simulink model "yukti_arduino_comms"  (R2025b)
settings: Solver=ode3  StartTime=0.0  StopTime=10  FixedStep=0.01  RelTol=1e-3  EnableMultiTasking=on
libraries: raspberrypiBasiclib x3, simulink_extras x2, instrumentseriallib x2, slpidlib x1, raspberrypiCommlib x1, raspberrypiNetworklib x1, instrumentlib x1
settings Model: FPTRunName=Active  ExtModeTrigDuration=2  Creator=YuktiVijay  LastModifiedBy=YuktiVijay
settings SolverCC: AlgebraicLoopSolver=TrustRegion  PositivePriorityOrder=on
settings DataIOCC: LimitDataPoints=on  SaveFormat=Array
settings OptimizationCC: ExpressionDepthLimit=2147483647.0  LifeSpan=Inf  MaxStackSize=200000
settings DebuggingCC: UnderspecifiedInitializationDetection=Classic  MergeDetectMultiDrivingBlocksExec=none  FcnCallInpInsideContextMsg=warning  UnconnectedInputMsg=warning  UnconnectedOutputMsg=warning  UnconnectedLineMsg=warning  AllowSymbolicDim=off  StateNameClashWarn=warning  SubsystemReferenceDiagnosticForUnitTest=warning  SFUnexpectedBacktrackingDiag=warning  SFNoUnconditionalDefaultTransitionDiag=warning  SFExecutionAtInitializationDiag=none  ArithmeticOperatorsInVariantConditions=warning
settings HardwareCC: ProdBitPerLong=64.0  ProdLargestAtomicInteger=LongLong  ProdLargestAtomicFloat=Double  ProdLongLongMode=on  ProdHWDeviceType=ARM Compatible->ARM Cortex-A (64-bit)  UseEmbeddedCoderFeatures=off  UseSimulinkCoderFeatures=off
settings ModelReferenceCC: EnableRefExpFcnMdlSchedulingChecks=on  PropagateSignalLabelsOutOfModel=off
settings SFSimCC: SimUseLocalCustomCode=off  CustomCodeUndefinedFunction=UseInterfaceOnly
settings RTWCC: SystemTargetFile=ert.tlc  HardwareBoard=Raspberry Pi (64bit)  TemplateMakefile=ert_default_tmf  GenerateReport=on  RTWVerbose=off  RTWUseLocalCustomCode=off  Toolchain=GNU GCC Embedded Linux  BuildConfiguration=Faster Runs  LaunchReport=on  GPUComputeCapability=3.5  Description=Embedded Coder
settings CodeAppCC: ForceParamTrailComments=on  OperatorAnnotations=on  StateflowObjectComments=on  MATLABSourceComments=on
settings ERTTargetCC: ExtModeTransport=2.0  ExtModeStaticAlloc=on  ExtModeMexFile=ext_xcp  ExtModeIntrfLevel=Level2 - Open  InlinedParameterPlacement=Hierarchical  DynamicArrayContainerType=coder::array  MultiwordLength=2048.0  ERTCustomFileBanners=off  SupportContinuousTime=on  SupportNonInlinedSFcns=on  RemoveResetFunc=off  SupportVariableSizeSignals=on  ModelStepFunctionPrototypeControlCompliant=off
settings ConfigComp: CovMetricSettings=dw  CovSaveCumulativeToWorkspaceVar=on  CovSaveSingleToWorkspaceVar=on  CovExternalEMLEnable=off  CovSFcnEnable=off

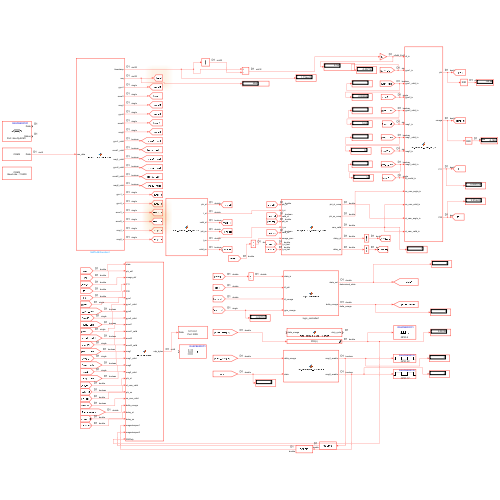
[thumbnail: Simulink's stored preview of the top-level diagram]
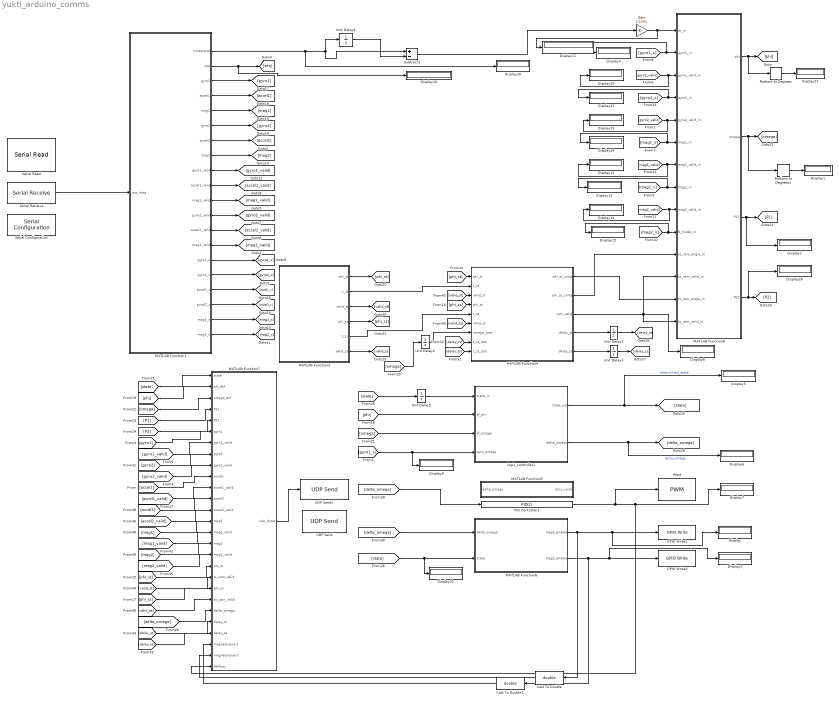
== system yukti_arduino_comms ==
  Cast To Double : DataTypeConversion  OutDataTypeStr=double  SaturateOnIntegerOverflow=off  RndMeth=Floor
  Cast To Double1 : DataTypeConversion  OutDataTypeStr=double  SaturateOnIntegerOverflow=off  RndMeth=Floor
  Display{,1..15,20..27} (24 alike) : Display
  GPIO Write1 : raspberrypiBasiclib/GPIO Write  BoardProperty=Pi 5 Model  gpio=22  blockPlatform=Raspberry Pi  PinNumber=17  board=[]  direction=[]
  GPIO Write3 : raspberrypiBasiclib/GPIO Write  BoardProperty=Pi 5 Model  gpio=17  blockPlatform=Raspberry Pi  PinNumber=17  board=[]  direction=[]
  Gain : Gain  Gain=1/1000
  MATLAB Function1 : MATLAB Function  TreatAsAtomicUnit=on
  MATLAB Function3 : MATLAB Function  TreatAsAtomicUnit=on
  MATLAB Function4 : MATLAB Function  TreatAsAtomicUnit=on
  MATLAB Function5 : MATLAB Function  TreatAsAtomicUnit=on
  MATLAB Function6 : MATLAB Function  TreatAsAtomicUnit=on
  MATLAB Function7 : MATLAB Function  TreatAsAtomicUnit=on
  MATLAB Function8 : MATLAB Function  TreatAsAtomicUnit=on
  PID Controller1 : slpidlib/PID Controller  Controller=PID  Form=Parallel  TimeDomain=Discrete-time  UseExternalTs=off  SampleTime=0.01  IntegratorMethod=Forward Euler  FilterMethod=Forward Euler  ControllerParametersSource=internal  P=0.001  I=0.0005  UseKiTs=on  D=0  UseExternalDerivativeSource=off  N=100  UseFilter=on  TunerSelectOption=Transfer Function Based (PID Tuner App)  InitialConditionSource=internal  InitialConditionForIntegrator=0.05  InitialConditionForFilter=0.05  DifferentiatorICPrevScaledInput=0  ExternalReset=none  TrackingMode=off  Kt=1  LimitOutput=on  SatLimitsSource=internal  UpperSaturationLimit=0.10  LowerSaturationLimit=0.05  LinearizeAsGain=on  AntiWindupMode=clamping  Kb=1  LimitIntegrator=off  UpperIntegratorSaturationLimit=inf  LowerIntegratorSaturationLimit=-inf  POutMin=[]  POutMax=[]  IOutMin=[]  IOutMax=[]  DOutMin=[]  DOutMax=[]  NOutMin=[]  NOutMax=[]  SumOutMin=[]  SumOutMax=[]  SaturationOutMin=[]  SaturationOutMax=[]  PParamMin=[]  PParamMax=[]  IParamMin=[]  IParamMax=[]  DParamMin=[]  DParamMax=[]  NParamMin=[]  NParamMax=[]  KbParamMin=[]  KbParamMax=[]  KtParamMin=[]  KtParamMax=[]  KbOutMin=[]  KbOutMax=[]  KtOutMin=[]  KtOutMax=[]  IntegratorOutMin=[]  IntegratorOutMax=[]  FilterOutMin=[]  FilterOutMax=[]  SumI1OutMin=[]  SumI1OutMax=[]  SumI2OutMin=[]  SumI2OutMax=[]  SumI3OutMin=[]  SumI3OutMax=[]  SumI4OutMin=[]  SumI4OutMax=[]  SumDOutMin=[]  SumDOutMax=[]  DifferentiatorOutMin=[]  DifferentiatorOutMax=[]  FilterDiffOutCoefMin=[]  FilterDiffOutCoefMax=[]  ReciprocalOutMin=[]  ReciprocalOutMax=[]  SumDenOutMin=[]  SumDenOutMax=[]  SumNumOutMin=[]  SumNumOutMax=[]  DivideOutMin=[]  DivideOutMax=[]  UdiffTsProdOutMin=[]  UdiffTsProdOutMax=[]  NTsProdOutMin=[]  NTsProdOutMax=[]  UintegralTsProdOutMin=[]  UintegralTsProdOutMax=[]  UngainTsProdOutMin=[]  UngainTsProdOutMax=[]  ClampingZeroOutDataTypeStr=Inherit: Inherit via back propagation  ClampingZeroOutMin=[]  ClampingZeroOutMax=[]  FilterDenConstantOutDataTypeStr=Inherit: Inherit via back propagation  FilterDenConstantOutMin=[]  FilterDenConstantOutMax=[]  PCopyOutDataTypeStr=Inherit: Inherit via back propagation  PCopyOutMin=[]  PCopyOutMax=[]  NCopyOutDataTypeStr=Inherit: Inherit via back propagation  NCopyOutMin=[]  NCopyOutMax=[]  IntegratorContinuousStateAttributes=''  IntegratorStateMustResolveToSignalObject=off  IntegratorRTWStateStorageClass=Auto  FilterContinuousStateAttributes=''  FilterStateMustResolveToSignalObject=off  FilterRTWStateStorageClass=Auto  ParallelPVariant=InternalParameters  IdealPVariant=Disabled  IVariant=InternalParameters  DVariant=InternalParameters  IntegratorVariant=Discrete  SatVariant=Enabled  AWVariant=DiscClampingParallel  PCopyVariant=Disabled  TRVariant=Disabled  FdbkBlocksVariant=Forward  IdealPFdbkVariant=Disabled  SatFdbkVariant=Disabled  DerivativeFilterVariant=ForwardEulerFilter  NVariant=InternalParameters  NCopyVariant=Disabled  FilterICVariant=InternalICsFilter  IntegratorICVariant=InternalICs  ExternalResetVariant=Disabled  TRSumVariant=Passthrough  SumFdbkVariant=Disabled  SumVariant=Sum_PID  TsampFilterVariant=InternalTs  TsampNgainVariant=Passthrough  TsampIntegralVariant=Disabled_SignalSpec  ExternalSaturationOutDataTypeStr=Inherit: Same as second input  DerivativeSourceVariant=ErrorSignal  PreIntVariant=InternalPreInt
  PWM : raspberrypiBasiclib/PWM  board=Pi 5 Model  Pin_=4  Frequency=500  blockPlatform=Raspberry Pi
  Radians to Degrees : simulink_extras/Transformations/Radians to Degrees
  Radians to Degrees1 : simulink_extras/Transformations/Radians to Degrees
  Serial Configuration : instrumentseriallib/Serial Configuration  Priority=-200000  PortSel=COM4  Port=COM4  ComPort=COM4  BaudRate=115200  DataBits=8  Parity=none  StopBits=1  ByteOrder=little-endian  FlowControl=none  Timeout=10  SimulateUsing=Interpreted execution  BlockInModel=on  aMode=1
  Serial Read : raspberrypiCommlib/Serial Read  board=Pi 5 Model  SCIModule_=/dev/ttyACM1  Baudrate_=115200  Parity=None  StopBits_=1  HardwareFlowControl=None  ByteOrder=LittleEndian  DataLength=62  DataType=uint8  OutputStatus=on  SampleTime=0.01  blockPlatform=RaspberryPi
  Serial Receive : instrumentseriallib/Serial Receive  Priority=1  PortSel=COM4  Port=COM4  ComPort=COM4  DataType=uint8  SaveDataType=uint8  ToggleHeader=on  Header=[85 170]  ToggleDataSize=on  DataSize=[1 172]  ToggleTerminator=off  Terminator=<none>  CustomTerminator=[]  InputFormat=Column major  EnableBlockingMode=on  ActionDataUnavailable=Output last received value  ActionWhenDataUnavailable=Output last received value  CustomValue=0  SampleTime=0.01  SimulateUsing=Interpreted execution  BlockInModel=on  aMode=1  LibraryInUse=instrumentlib
  Subtract1 : Sum  Inputs=+-
  UDP Send : raspberrypiNetworklib/UDP Send  remoteURL='255.255.255.255'  remotePort=25000  localURL='0.0.0.0'  localPortSource=Automatically determine  localPort=-1  sampletime=-1  blockPlatform=Raspberry Pi  separateLengthPort=0
  UDP Send1 : instrumentlib/UDP Send  Host=127.0.0.1  Port=5005  LocalAddress=0.0.0.0  LocalPort=-1  EnablePortSharing=off  OutputDatagramPacketSize=280  ByteOrder=little-endian  EnableBlockingMode=on  SimulateUsing=Interpreted execution
  Unit Delay{1..5} (5 alike) : UnitDelay  SampleTime=-1  HasFrameUpgradeWarning=on
  logic_controller1 : MATLAB Function  TreatAsAtomicUnit=on
  wires:
  [gyro1_x] -> Display4/1, MATLAB Function8/2(gyro1_in)
  [mag1_x] -> Display24/1, MATLAB Function8/6(mag1_in)
  MATLAB Function1/20(mag2_x) -> [mag2_x]
  MATLAB Function1/19(mag1_x) -> [mag1_x]
  Unit Delay2/1 -> MATLAB Function4/7(omega_prev)
  MATLAB Function3/2(t_st) -> MATLAB Function4/2(t_st)
  MATLAB Function3/5(t_ss) -> MATLAB Function4/5(t_ss)
  MATLAB Function4/4(delay_st) -> Unit Delay1/1
  MATLAB Function4/5(delay_ss) -> Unit Delay3/1
  Unit Delay4/1 -> Subtract1/2
  MATLAB Function1/1(timestamp) -> Display20/1, Unit Delay4/1, Subtract1/1
  Subtract1/1 -> Gain/1
  MATLAB Function4/1(phi_st_comp) -> MATLAB Function8/13(st_cam_angle_in)
  MATLAB Function4/3(cam_valid) -> MATLAB Function8/14(st_cam_valid_in), Display8/1, MATLAB Function8/12(ss_cam_valid_in)
  [gyro1_x] -> Display9/1, logic_controller1/4(gyro_omega)
  Unit Delay5/1 -> logic_controller1/1(state_in)
  Gain/1 -> Display11/1, MATLAB Function8/1(dt_in)
  [gyro1] -> MATLAB Function7/6(gyro1)
  MATLAB Function1/15(gyro1_x) -> [gyro1_x]
  MATLAB Function1/16(gyro2_x) -> [gyro2_x]
  MATLAB Function1/11(mag1_valid) -> [mag1_valid]
  MATLAB Function1/9(gyro1_valid) -> [gyro1_valid]
  MATLAB Function1/10(accel1_valid) -> [accel1_valid]
  MATLAB Function1/12(gyro2_valid) -> [gyro2_valid]
  MATLAB Function1/13(accel2_valid) -> [accel2_valid]
  MATLAB Function1/14(mag2_valid) -> [mag2_valid]
  MATLAB Function1/3(gyro1) -> [gyro1]
  MATLAB Function1/4(accel1) -> [accel1]
  MATLAB Function1/5(mag1) -> [mag1]
  MATLAB Function1/6(gyro2) -> [gyro2]
  MATLAB Function1/7(accel2) -> [accel2]
  MATLAB Function1/8(mag2) -> [mag2]
  MATLAB Function1/2(seq) -> Display10/1, [seq]
  MATLAB Function1/17(accel1_x) -> [accel1_x]
  MATLAB Function1/18(accel2_x) -> [accel2_x]
  [gyro1_valid] -> Display25/1, MATLAB Function8/3(gyro1_valid_in)
  [mag2_x] -> Display13/1, MATLAB Function8/8(mag2_in)
  [mag2_x] -> Display15/1, MATLAB Function8/10(B_model_in)
  MATLAB Function4/2(phi_ss_comp) -> MATLAB Function8/11(ss_cam_angle_in)
  [mag2_valid] -> Display14/1, MATLAB Function8/9(mag2_valid_in)
  [mag1_valid] -> Display12/1, MATLAB Function8/7(mag1_valid_in)
  [gyro2_valid] -> Display23/1, MATLAB Function8/5(gyro2_valid_in)
  MATLAB Function3/1(phi_st) -> [phi_st]
  [phi_st] -> MATLAB Function4/1(phi_st)
  [phi_st] -> MATLAB Function7/18(phi_st)
  MATLAB Function3/4(phi_ss) -> [phi_ss]
  [phi_ss] -> MATLAB Function4/4(phi_ss)
  [phi_ss] -> MATLAB Function7/20(phi_ss)
  MATLAB Function8/1(phi) -> Radians to Degrees/1, [phi]
  [phi] -> logic_controller1/2(kf_phi)
  [phi] -> MATLAB Function7/2(phi_ekf)
  [omega] -> Unit Delay2/1
  [omega] -> logic_controller1/3(kf_omega)
  [omega] -> MATLAB Function7/3(omega_ekf)
  MATLAB Function8/4(P22) -> Display26/1, [P2]
  [P1] -> MATLAB Function7/4(P11)
  [P2] -> MATLAB Function7/5(P22)
  logic_controller1/1(state_out) -> Display5/1, [state]  "determined_state"
  [state] -> Unit Delay5/1
  [state] -> Display22/1, MATLAB Function6/2(state)
  logic_controller1/2(delta_omega) -> Display6/1, [delta_omega]  "delta_omega"
  [state] -> MATLAB Function7/1(state)
  [delta_omega] -> MATLAB Function7/22(delta_omega)
  [delta_omega] -> MATLAB Function6/1(delta_omega)
  Unit Delay3/1 -> [delay_ss]
  [delay_ss] -> MATLAB Function4/9(t_ss_last)
  [delay_st] -> MATLAB Function4/8(t_st_last)
  Unit Delay1/1 -> [delay_st]
  [delay_st] -> MATLAB Function7/23(delay_st)
  [delay_ss] -> MATLAB Function7/24(delay_ss)
  [accel2_valid] -> MATLAB Function7/13(accel2_valid)
  [mag2_valid] -> MATLAB Function7/17(mag2_valid)
  [mag1_valid] -> MATLAB Function7/15(mag1_valid)
  [accel1_valid] -> MATLAB Function7/11(accel1_valid)
  [accel2] -> MATLAB Function7/12(accel2)
  [accel1] -> MATLAB Function7/10(accel1)
  [gyro2] -> MATLAB Function7/8(gyro2)
  [mag1] -> MATLAB Function7/14(mag1)
  [gyro1_valid] -> MATLAB Function7/7(gyro1_valid)
  [gyro2_valid] -> MATLAB Function7/9(gyro2_valid)
  [mag2] -> MATLAB Function7/16(mag2)
  MATLAB Function3/6(valid_ss) -> [valid_ss]
  MATLAB Function3/3(valid_st) -> [valid_st]
  [valid_st] -> MATLAB Function4/3(valid_st)
  [valid_ss] -> MATLAB Function4/6(valid_ss)
  [valid_ss] -> MATLAB Function7/21(ss_cam_valid)
  [valid_st] -> MATLAB Function7/19(st_cam_valid)
  Serial Receive/1 -> MATLAB Function1/1(raw_data)
  MATLAB Function8/3(P11) -> Display2/1, [P1]
  [gyro2_x] -> Display21/1, MATLAB Function8/4(gyro2_in)
  Radians to Degrees/1 -> Display27/1
  Radians to Degrees1/1 -> Display1/1
  MATLAB Function8/2(omega) -> Radians to Degrees1/1, [omega]
  MATLAB Function7/1(udp_bytes) -> UDP Send1/1
  MATLAB Function6/1(mag1_enable) -> Display/1, GPIO Write1/1, Cast To Double/1
  MATLAB Function6/2(mag2_enable) -> Cast To Double1/1, Display3/1, GPIO Write3/1
  PID Controller1/1 -> MATLAB Function7/27(RWDuty), Display7/1, PWM/1
  [delta_omega] -> PID Controller1/1
  Cast To Double/1 -> MATLAB Function7/26(magnetorquer2)
  Cast To Double1/1 -> MATLAB Function7/25(magnetorquer1)

== matlab function yukti_arduino_comms/MATLAB Function5 ==
  data: delta_omega input; duty_cycle output
function duty_cycle = map_delta_omega_to_pwm(delta_omega)
%#codegen
% Simple mapping: delta_omega to duty cycle
% Positive delta_omega = speed up spacecraft = slow down wheel (less throttle)
% Negative delta_omega = slow down spacecraft = speed up wheel (more throttle)

    persistent current_duty;
    
    if isempty(current_duty)
        current_duty = 0.05;  % Start at minimum throttle
    end
    
    % Gain: how much duty cycle changes per rad/s of delta_omega
    gain = 0.01;  % Tune this
    
    % Update duty cycle
    current_duty = current_duty - gain * delta_omega;
    
    % Clamp to valid range
    current_duty = max(0.05, min(0.10, current_duty));
    
    duty_cycle = current_duty;

end

== matlab function yukti_arduino_comms/MATLAB Function6 ==
  data: delta_omega input; mag1_enable output; state input; mag2_enable output
function [mag1_enable, mag2_enable] = magnetorquer_command(delta_omega, state)
%#codegen
% PLACEHOLDER: Converts delta_omega to magnetorquer GPIO commands
%
% Inputs:
%   delta_omega - desired change in angular velocity
%   state - current controller state (0=detumble uses mags)
%
% Outputs:
%   mag1_enable - GPIO signals for magnetorquer 1
%   mag2_enable - GPIO signals for magnetorquer 2
%   Not sure about direction of spin, try if it speeds up instead: delta_omega > 0.01  
%
    mag1_enable = false;
    mag2_enable = false;
    
    if state == 0
        if delta_omega < -0.01  % Need to slow down
            mag1_enable = true;
            mag2_enable = true;
        end
    end
end

== matlab function yukti_arduino_comms/MATLAB Function7 ==
  data: udp_bytes output; state input; phi_ekf input; omega_ekf input; P11 input; P22 input; gyro1 input; gyro1_valid input; gyro2 input; gyro2_valid input; accel1 input; accel1_valid input; accel2 input; accel2_valid input; mag1 input; mag1_valid input; mag2 input; mag2_valid input; phi_st input; st_cam_valid input; phi_ss input; ss_cam_valid input; delta_omega input; delay_st input; delay_ss input; magnetorquer1 input; magnetorquer2 input; RWDuty input
function udp_bytes = pack_telemetry(state, phi_ekf, omega_ekf, P11, P22, ...
                                     gyro1, gyro1_valid, ...
                                     gyro2, gyro2_valid, ...
                                     accel1, accel1_valid, ...
                                     accel2, accel2_valid, ...
                                     mag1, mag1_valid, ...
                                     mag2, mag2_valid, ...
                                     phi_st, st_cam_valid, ...
                                     phi_ss, ss_cam_valid, ...
                                     delta_omega, delay_st, delay_ss, magnetorquer1,magnetorquer2,RWDuty)
%#codegen
% Packs all telemetry into byte array for UDP transmission
% Get timestamp internally
    timestamp = get_unix_time();

% Pack validity flags into single double as bitmask
% Bit 0: gyro1_valid
% Bit 1: gyro2_valid
% Bit 2: accel1_valid
% Bit 3: accel2_valid
% Bit 4: mag1_valid
% Bit 5: mag2_valid
% Bit 6: ss_cam_valid
% Bit 7: st_cam_valid
    validity_flags = double(0);
    if gyro1_valid,   validity_flags = validity_flags + 1;   end
    if gyro2_valid,   validity_flags = validity_flags + 2;   end
    if accel1_valid,  validity_flags = validity_flags + 4;   end
    if accel2_valid,  validity_flags = validity_flags + 8;   end
    if mag1_valid,    validity_flags = validity_flags + 16;  end
    if mag2_valid,    validity_flags = validity_flags + 32;  end
    if ss_cam_valid,  validity_flags = validity_flags + 64;  end
    if st_cam_valid,  validity_flags = validity_flags + 128; end

% Total: 35 doubles = 280 bytes
    num_doubles = 35;

% Pack all values into double array
    data = zeros(1, num_doubles);
    data(1) = timestamp;
    data(2) = double(state);
    data(3) = phi_ekf*57.2957795131;
    data(4) = omega_ekf*57.2957795131;
    data(5) = P11;
    data(6) = P22;
    data(7) = gyro1(1)*57.2957795131;
    data(8) = gyro1(2)*57.2957795131;
    data(9) = gyro1(3)*57.2957795131;
    data(10) = gyro2(1)*57.2957795131;
    data(11) = gyro2(2)*57.2957795131;
    data(12) = gyro2(3)*57.2957795131;
    data(13) = accel1(1);
    data(14) = accel1(2);
    data(15) = accel1(3);
    data(16) = accel2(1);
    data(17) = accel2(2);
    data(18) = accel2(3);
    data(19) = mag1(1);
    data(20) = mag1(2);
    data(21) = mag1(3);
    data(22) = mag2(1);
    data(23) = mag2(2);
    data(24) = mag2(3);
    data(25) = phi_st*57.2957795131;
    data(26) = phi_ss*57.2957795131;
    data(27) = delta_omega*57.2957795131;
    data(28) = delay_st;
    data(29) = delay_ss;
    data(30) = validity_flags;
    data(31) = double(magnetorquer1);
    data(32) = double(magnetorquer2);
    data(33) = RWDuty;
    data(34) = 0;  % reserved
    data(35) = 0;  % reserved

% Convert to bytes
    udp_bytes = typecast(data, 'uint8');
end

== matlab function yukti_arduino_comms/MATLAB Function3 ==
  data: phi_st output; t_st output; valid_st output; phi_ss output; t_ss output; valid_ss output
function [phi_st, t_st, valid_st, phi_ss, t_ss, valid_ss] = load_camera_bin_wrapper()
    [phi_st, t_st, valid_st, phi_ss, t_ss, valid_ss] = load_camera_bin();
end

== matlab function yukti_arduino_comms/MATLAB Function1 ==
  data: timestamp output; seq output; gyro1 output; raw_data input; accel1 output; mag1 output; gyro2 output; accel2 output; mag2 output; gyro1_valid output; accel1_valid output; mag1_valid output; gyro2_valid output; accel2_valid output; mag2_valid output; gyro1_x output; gyro2_x output; accel1_x output; accel2_x output; mag1_x output; mag2_x output
function [timestamp, seq, gyro1, accel1, mag1, gyro2, accel2, mag2, ...
          gyro1_valid, accel1_valid, mag1_valid, gyro2_valid, accel2_valid, mag2_valid, ...
          gyro1_x, gyro2_x, accel1_x, accel2_x, mag1_x, mag2_x] = Parse_Arduino_Packet(raw_data) %#codegen
    % Parse 86-byte binary packet from Arduino dual ICM-20948 setup
    %
    % Packet structure:
    % [0-1]   Header: 0x55, 0xAA
    % [2]     Validity flags (6 bits)
    % [3]     Reserved
    % [4-7]   Sequence number (uint32, little-endian)
    % [8-11]  Timestamp (uint32, little-endian)
    % [12-23] Gyro1 XYZ (3 floats)
    % [24-35] Accel1 XYZ (3 floats)
    % [36-47] Mag1 XYZ (3 floats)
    % [48-59] Gyro2 XYZ (3 floats)
    % [60-71] Accel2 XYZ (3 floats)
    % [72-83] Mag2 XYZ (3 floats)
    % [84-85] CRC16-CCITT

    PACKET_SIZE = 86;
    
    % Initialize outputs
    gyro1 = zeros(3, 1, 'single');
    accel1 = zeros(3, 1, 'single');
    mag1 = zeros(3, 1, 'single');
    gyro2 = zeros(3, 1, 'single');
    accel2 = zeros(3, 1, 'single');
    mag2 = zeros(3, 1, 'single');
    
    seq = uint32(0);
    timestamp = uint32(0);
    
    % Individual validity flags
    gyro1_valid = false;
    accel1_valid = false;
    mag1_valid = false;
    gyro2_valid = false;
    accel2_valid = false;
    mag2_valid = false;
    
    % X-axis values
    gyro1_x = single(0);
    gyro2_x = single(0);
    accel1_x = single(0);
    accel2_x = single(0);
    mag1_x = single(0);
    mag2_x = single(0);

    % Search for header (0x55, 0xAA) in the data stream
    header_found = false;
    start_idx = 1;
    
    for i = 1:(length(raw_data) - 1)
        if raw_data(i) == uint8(85) && raw_data(i+1) == uint8(170)  % 0x55, 0xAA
            % Check if we have enough bytes for a complete packet
            if (i + PACKET_SIZE - 1) <= length(raw_data)
                start_idx = i;
                header_found = true;
                break;
            end
        end
    end
    
    if ~header_found
        return;
    end
    
    % Extract the packet
    packet = raw_data(start_idx:(start_idx + PACKET_SIZE - 1));
    
    % Verify CRC (CRC is over bytes 1-84, CRC stored in bytes 85-86)
    crc_received = uint16(packet(85)) + bitshift(uint16(packet(86)), 8);
    crc_calculated = crc16_ccitt(packet(1:84));
    
    if crc_received ~= crc_calculated
        return;
    end
    
    % Parse validity flags (byte 3)
    validity_byte = packet(3);
    gyro1_valid  = bitand(validity_byte, uint8(1)) ~= 0;
    accel1_valid = bitand(validity_byte, uint8(2)) ~= 0;
    mag1_valid   = bitand(validity_byte, uint8(4)) ~= 0;
    gyro2_valid  = bitand(validity_byte, uint8(8)) ~= 0;
    accel2_valid = bitand(validity_byte, uint8(16)) ~= 0;
    mag2_valid   = bitand(validity_byte, uint8(32)) ~= 0;
    
    % Parse sequence number (bytes 5-8, little-endian uint32)
    seq = uint32(packet(5)) + ...
          bitshift(uint32(packet(6)), 8) + ...
          bitshift(uint32(packet(7)), 16) + ...
          bitshift(uint32(packet(8)), 24);
    
    % Parse timestamp (bytes 9-12, little-endian uint32)
    timestamp = uint32(packet(9)) + ...
                bitshift(uint32(packet(10)), 8) + ...
                bitshift(uint32(packet(11)), 16) + ...
                bitshift(uint32(packet(12)), 24);
    
    % Parse 18 floats (72 bytes total, starting at byte 13)
    floats = zeros(18, 1, 'single');
    for i = 1:18
        byte_offset = 12 + (i - 1) * 4;  % Starts at byte 13 (index 13)
        bytes = uint8([packet(byte_offset + 1), ...
                       packet(byte_offset + 2), ...
                       packet(byte_offset + 3), ...
                       packet(byte_offset + 4)]);
        floats(i) = typecast(bytes, 'single');
    end
    
    % Extract sensor data vectors
    gyro1  = floats(1:3);    % Bytes 13-24
    accel1 = floats(4:6);    % Bytes 25-36
    mag1   = floats(7:9);    % Bytes 37-48
    gyro2  = floats(10:12);  % Bytes 49-60
    accel2 = floats(13:15);  % Bytes 61-72
    mag2   = floats(16:18);  % Bytes 73-84
    
    % Extract x-axis values
    gyro1_x  = floats(1);
    accel1_x = floats(4);
    mag1_x   = floats(7);
    gyro2_x  = floats(10);
    accel2_x = floats(13);
    mag2_x   = floats(16);
end

function crc = crc16_ccitt(data)
    crc = uint16(65535);  % 0xFFFF
    for i = 1:length(data)
        crc = bitxor(crc, bitshift(uint16(data(i)), 8));
        for j = 1:8
            if bitand(crc, uint16(32768)) ~= uint16(0)  % 0x8000
                crc = bitxor(bitshift(crc, 1), uint16(4129));  % 0x1021
            else
                crc = bitshift(crc, 1);
            end
        end
    end
    crc = bitand(crc, uint16(65535));
end

== matlab function yukti_arduino_comms/logic_controller1 ==
  data: state_in input; kf_phi input; kf_omega input; gyro_omega input; state_out output; delta_omega output
function [state_out,delta_omega] = logic_controller(state_in,kf_phi,kf_omega,gyro_omega)

    % State controller parameters
    omega_detumble_target = 0.1*pi; % Target slew rate for detumble phase
    phi_starfield_min = -3*pi/4; % S/C attitude minimum to see star field
    phi_starfield_max = -pi/4; % S/C attitude maximum to see star field
    omega_slowrotation_target = 0.02*pi; % Target slew rate for slowrotation phase
    phi_mars = -5*pi/8; % Position of mars
    phi_mars_delta = pi/32; % Field of view tolerance for imaging mars
    omega_imaging_target = omega_slowrotation_target; % Maximum slew rate allowable for science imaging

    % By default, assume state_out = state_in and no actions are to be
    % taken
    state_out = state_in;
    delta_omega = 0;
    gyro_omega = double(gyro_omega);

    % S0: Detubmble
    if state_in == 0
        
        % Read gyro output directly
        omega = gyro_omega;
        
        % Check if we have achieved the goal for this state: sufficiently
        % slow rotation
        if abs(omega) < omega_detumble_target

            state_out = 1;
        
        % If not, proceed    
        else

            % Set delta_omega to try and null out spin
            delta_omega = -omega;


        end
    
    
    
    % S1: Slow rotation / coarse pointing
    elseif state_in == 1

        % Read from kalman filter
        phi = kf_phi;
        omega = kf_omega;

        % Check if we have achieved the goal for this state: very slow rotation, and
        % visibility of the star field
        omega_requirement = abs(omega) < omega_slowrotation_target;
        phi_requirement = phi > phi_starfield_min && phi < phi_starfield_max;

        % If so, move to next state
        if omega_requirement && phi_requirement

            state_out = 2;

        % If not, proceed with this state
        else
            
            % Check if we need to move back to S0
            if abs(omega) > omega_detumble_target 

                state_out = 0;
        
            % We are either spinning too fast, or not within the right
            % attitude range. First, if we are within the attitude range,
            % try to null out spin
            elseif phi_requirement

                delta_omega = -kf_omega;
            
            % If we are not within the
            % desired attitude range, then try to spin in the direction we
            % are already going at 2x omega_slowrotation_target
            else
                
                if omega>0

                    delta_omega = 2*omega_slowrotation_target - omega;

                else

                    delta_omega = - (2*omega_slowrotation_target - abs(omega));
                
                end

            end

        end

    % S3: Fine Pointing
    elseif state_in == 2
    
        % Read from kalman filter
        phi = kf_phi;
        omega = kf_omega;

        % Check if we have achieved the goal for this state: pointing at
        % Mars within FOV bounds, with slow enough rotation for imaging
        phi_requirement = phi > phi_mars-phi_mars_delta && phi < phi_mars + phi_mars_delta;
        omega_requirement = abs(omega) < omega_imaging_target;
        
        % If so, move to next state
        if phi_requirement && omega_requirement
            
            state_out = 3;

        % If not, proceed with this state
        else

            % First, check if we need to bump back up to S1, if we have
            % started spinning too fast or left the starfield
            if phi < phi_starfield_min || phi > phi_starfield_max || abs(omega) > 5*omega_slowrotation_target

                state_out = 1;
            
            % Getting to this stage means we are viewing the starfield,
            % spinning relatively slowly. Therefore, slew towards Mars

            % Our slew rate will depend on how far we are from the desired
            % attitude window.
            elseif phi-phi_mars > 5*phi_mars_delta

                delta_omega =  - (omega_slowrotation_target + omega);

            elseif phi-phi_mars < 5*phi_mars_delta

                delta_omega = (omega_slowrotation_target + omega);

             elseif phi-phi_mars > 2*phi_mars_delta

                delta_omega =  - (omega_slowrotation_target/2 + omega);

            elseif phi-phi_mars < 2*phi_mars_delta

                delta_omega = (omega_slowrotation_target/2 + omega);

           % Finally, if we are within the attitude range, null out
           % velocity
            elseif abs(phi-phi_mars) < phi_mars_delta

                delta_omega = -omega;

            end
                
    end
    
end

== matlab function yukti_arduino_comms/MATLAB Function8 ==
  data: dt_in input; phi output; gyro1_in input; gyro1_valid_in input; gyro2_in input; gyro2_valid_in input; mag1_in input; mag1_valid_in input; mag2_in input; mag2_valid_in input; B_model_in input; omega output; P11 output; P22 output; ss_cam_angle_in input; ss_cam_valid_in input; st_cam_angle_in input; st_cam_valid_in input
function [phi, omega, P11, P22] = ekf_attitude_step_async(dt_in, ...
                                                      gyro1_in, gyro1_valid_in, ...
                                                      gyro2_in, gyro2_valid_in, ...
                                                      mag1_in, mag1_valid_in, ...
                                                      mag2_in, mag2_valid_in, ...
                                                      B_model_in, ...
                                                      ss_cam_angle_in, ss_cam_valid_in, ...
                                                      st_cam_angle_in, st_cam_valid_in)
% Implements one step of an asynchronous EKF for 1D Attitude.
% This function MUST be called at the rate of the FASTEST sensor (e.g., Gyro).
%
% PREDICTION is run every time.
% UPDATE is run sequentially for each sensor group *only if* its 
% corresponding 'valid' flag is true.
%
% Outputs:
%   phi   - estimated angle (rad)
%   omega - estimated angular velocity (rad/s)
%   P11   - angle variance
%   P22   - angular velocity variance

%#codegen

% --- Define Persistent Variables ---
persistent x_hat P is_initialized;

% --- Initialization (Runs only once) ---
if isempty(is_initialized)
    x_hat = zeros(2, 1, 'double'); % [rad; rad/s]
    P = diag([(10*pi/180)^2, (5*pi/180)^2]); 
    is_initialized = true;
end

% --- Filter Constants ---
% State definition: x_hat = [angle; angular_velocity]

% --- Defensive casting of inputs to fixed types / sizes for codegen ---
dt      = double(dt_in);
gyro1   = double(gyro1_in);
gyro2   = double(gyro2_in);
mag1    = double(mag1_in);
mag2    = double(mag2_in);
B_model = double(B_model_in);
ss_cam  = double(ss_cam_angle_in);
st_cam  = double(st_cam_angle_in);

% Ensure scalars: if arrays are passed, take first element (defensive)
if numel(dt) > 1,      dt = dt(1);           end
if numel(gyro1) > 1,   gyro1 = gyro1(1);     end
if numel(gyro2) > 1,   gyro2 = gyro2(1);     end
if numel(mag1) > 1,    mag1 = mag1(1);       end
if numel(mag2) > 1,    mag2 = mag2(1);       end
if numel(B_model) > 1, B_model = B_model(1); end
if numel(ss_cam) > 1,  ss_cam = ss_cam(1);   end
if numel(st_cam) > 1,  st_cam = st_cam(1);   end

% Cast valid flags to logical scalars for deterministic codegen branching
gyro1_valid  = logical(gyro1_valid_in);
gyro2_valid  = logical(gyro2_valid_in);
mag1_valid   = logical(mag1_valid_in);
mag2_valid   = logical(mag2_valid_in);
ss_cam_valid = logical(ss_cam_valid_in);
st_cam_valid = logical(st_cam_valid_in);

% Noise STDs
noiseSTDSystem = (1 * pi / 180); % rad/s^2 (Process noise)
noiseSTDGyroMeasurement1 = (1 * pi / 180); % rad (Gyro1)
noiseSTDGyroMeasurement2 = (1 * pi / 180); % rad (Gyro2)
noiseSTDMagMeasurement1 = (5); % nT (Mag1)
noiseSTDMagMeasurement2 = (6); % nT (Mag2)
noiseSTDSsCam = (1 * pi / 180); % rad (Sun Sensor)
noiseSTDStCam = (1 * pi / 180); % rad (Star Tracker)

% Magnetometer orientations
magAngle1 = 0;       % rad
magAngle2 = pi / 2;  % rad

% State transition matrix
F = [1, dt; 
     0, 1];

% Process Noise Covariance (Q)
L = [0; dt];
q_val = noiseSTDSystem^2;
Q = L * q_val * L'; 

% Measurement Noise Covariances (R) - split by sensor
R_gyro1 = noiseSTDGyroMeasurement1^2; % 1x1
R_gyro2 = noiseSTDGyroMeasurement2^2; % 1x1

R_mag1 = noiseSTDMagMeasurement1^2; % 1x1
R_mag2 = noiseSTDMagMeasurement2^2; % 1x1

R_ss_cam = noiseSTDSsCam^2; % 1x1
R_st_cam = noiseSTDStCam^2; % 1x1
              
% State size
sizeF = 2;

% =========================================================
% --- 1. EKF PREDICTION STEP (Time Update) ---
% =========================================================
x_hat = F * x_hat; 
P = F * P * F' + Q;

% =========================================================
% --- 2. EKF UPDATE STEP (Measurement Updates) ---
% =========================================================

% --- GYRO1 UPDATE ---
if gyro1_valid
    z_gyro1 = gyro1;
    h_gyro1 = x_hat(2);
    H_gyro1 = [0, 1];
    S_gyro1 = H_gyro1 * P * H_gyro1' + R_gyro1;
    PH_transpose = P * H_gyro1';
    K_gyro1 = PH_transpose * (1.0 / S_gyro1);
    innovation_gyro1 = z_gyro1 - h_gyro1;
    x_hat = x_hat + K_gyro1 * innovation_gyro1;
    I_KH = (eye(sizeF) - K_gyro1 * H_gyro1);
    P = I_KH * P * I_KH' + K_gyro1 * R_gyro1 * K_gyro1';
end

% --- GYRO2 UPDATE ---
if gyro2_valid
    z_gyro2 = gyro2;
    h_gyro2 = x_hat(2);
    H_gyro2 = [0, 1];
    S_gyro2 = H_gyro2 * P * H_gyro2' + R_gyro2;
    PH_transpose = P * H_gyro2';
    K_gyro2 = PH_transpose * (1.0 / S_gyro2);
    innovation_gyro2 = z_gyro2 - h_gyro2;
    x_hat = x_hat + K_gyro2 * innovation_gyro2;
    I_KH = (eye(sizeF) - K_gyro2 * H_gyro2);
    P = I_KH * P * I_KH' + K_gyro2 * R_gyro2 * K_gyro2';
end

% --- MAGNETOMETER 1 UPDATE ---
if mag1_valid
    z_mag1 = mag1;
    h_mag1 = cos(x_hat(1) + magAngle1) * B_model;
    H_mag1 = [-sin(x_hat(1) + magAngle1) * B_model, 0];
    S_mag1 = H_mag1 * P * H_mag1' + R_mag1;
    PH_transpose = P * H_mag1';
    K_mag1 = PH_transpose * (1.0 / S_mag1);
    innovation_mag1 = z_mag1 - h_mag1;
    x_hat = x_hat + K_mag1 * innovation_mag1;
    I_KH = (eye(sizeF) - K_mag1 * H_mag1);
    P = I_KH * P * I_KH' + K_mag1 * R_mag1 * K_mag1';
end

% --- MAGNETOMETER 2 UPDATE ---
if mag2_valid
    z_mag2 = mag2;
    h_mag2 = cos(x_hat(1) + magAngle2) * B_model;
    H_mag2 = [-sin(x_hat(1) + magAngle2) * B_model, 0];
    S_mag2 = H_mag2 * P * H_mag2' + R_mag2;
    PH_transpose = P * H_mag2';
    K_mag2 = PH_transpose * (1.0 / S_mag2);
    innovation_mag2 = z_mag2 - h_mag2;
    x_hat = x_hat + K_mag2 * innovation_mag2;
    I_KH = (eye(sizeF) - K_mag2 * H_mag2);
    P = I_KH * P * I_KH' + K_mag2 * R_mag2 * K_mag2';
end

% --- SUN SENSOR UPDATE ---
if ss_cam_valid
    z_ss_cam = ss_cam;
    h_ss_cam = x_hat(1);
    H_ss_cam = [1, 0];
    S_ss_cam = H_ss_cam * P * H_ss_cam' + R_ss_cam;
    PH_transpose = P * H_ss_cam';
    K_ss_cam = PH_transpose * (1.0 / S_ss_cam);
    innovation_ss_cam = z_ss_cam - h_ss_cam;
    innovation_ss_cam = wrapToPi(innovation_ss_cam);
    x_hat = x_hat + K_ss_cam * innovation_ss_cam;
    I_KH = (eye(sizeF) - K_ss_cam * H_ss_cam);
    P = I_KH * P * I_KH' + K_ss_cam * R_ss_cam * K_ss_cam';
end

% --- STAR TRACKER UPDATE ---
if st_cam_valid
    z_st_cam = st_cam;
    h_st_cam = x_hat(1);
    H_st_cam = [1, 0];
    S_st_cam = H_st_cam * P * H_st_cam' + R_st_cam;
    PH_transpose = P * H_st_cam';
    K_st_cam = PH_transpose * (1.0 / S_st_cam);
    innovation_st_cam = z_st_cam - h_st_cam;
    innovation_st_cam = wrapToPi(innovation_st_cam);
    x_hat = x_hat + K_st_cam * innovation_st_cam;
    I_KH = (eye(sizeF) - K_st_cam * H_st_cam);
    P = I_KH * P * I_KH' + K_st_cam * R_st_cam * K_st_cam';
end

% --- Final Angle Wrap ---
x_hat(1) = wrapToPi(x_hat(1));

% --- Set Outputs (split) ---
phi = x_hat(1);
omega = x_hat(2);
P11 = P(1,1);
P22 = P(2,2);

end

% ----------------------------
% Local helper functions
% ----------------------------
function ang = wrapToPi(a)
    ang = a - 2.0 * pi * floor((a + pi) / (2.0 * pi));
end

== matlab function yukti_arduino_comms/MATLAB Function4 ==
  data: phi_st input; phi_st_comp output; t_st input; valid_st input; phi_ss input; t_ss input; valid_ss input; omega_prev input; t_st_last input; t_ss_last input; phi_ss_comp output; cam_valid output; delay_st output; delay_ss output
function [phi_st_comp, phi_ss_comp, cam_valid, delay_st, delay_ss] = ...
    compensate_camera_delay(phi_st, t_st, valid_st, phi_ss, t_ss, valid_ss, omega_prev, t_st_last, t_ss_last)
%#codegen
% Compensates camera measurements for time delay
% Only marks valid if timestamp is newer than last used
%
% Inputs:
%   phi_st, t_st, valid_st - star tracker angle, timestamp, file valid
%   phi_ss, t_ss, valid_ss - sun sensor angle, timestamp, file valid
%   omega_prev - previous omega estimate from EKF (rad/s)
%   t_st_last - last used star tracker timestamp
%   t_ss_last - last used sun sensor timestamp
%
% Outputs:
%   phi_st_comp, phi_ss_comp - delay-compensated angles
%   cam_valid - true if at least one camera has NEW data
%   delay_st, delay_ss - measured delays (for telemetry)

    % Get current time
    t_now = get_unix_time();
    
    % Initialize outputs
    phi_st_comp = 0;
    phi_ss_comp = 0;
    delay_st = 0;
    delay_ss = 0;
    cam_valid = 0;

    
    % Star tracker compensation
    st_new = valid_st && (t_st > t_st_last);
    if st_new
        delay_st = t_now - t_st;
        phi_st_comp = phi_st + omega_prev * delay_st;
        phi_st_comp = wrapToPi(phi_st_comp);
    end
    
    % Sun sensor compensation
    ss_new = valid_ss && (t_ss > t_ss_last);
    if ss_new
        delay_ss = t_now - t_ss;
        phi_ss_comp = phi_ss + omega_prev * delay_ss;
        phi_ss_comp = wrapToPi(phi_ss_comp);
    end
    
    % Valid if either camera has new data
    if st_new || ss_new
        cam_valid = 1;
    else
        cam_valid = 0;
    end
end

function ang = wrapToPi(a)
    ang = a - 2*pi * floor((a + pi) / (2*pi));
end
